simulink model "Model1"  (R2015b)
settings: Solver=ode45  StartTime=0.0  StopTime=4  RelTol=1e-6
undefined symbols (not defined in the file): B_f, B_w, g, J_f, J_w, l_f, l_w, m_f, m_w
settings Model: Creator=USUARIO  LastModifiedBy=USUARIO
settings DataIOCC: LimitDataPoints=off  SaveFormat=Array
settings DebuggingCC: SolverPrmCheckMsg=warning
settings HardwareCC: ProdBitPerPointer=32  ProdLargestAtomicFloat=None  ProdIntDivRoundTo=Undefined  ProdEndianess=Unspecified  ProdWordSize=32  ProdHWDeviceType=32-bit Generic
settings GRTTargetCC: GeneratePreprocessorConditionals=Disable all
settings ConfigComp: CovModelRefEnable=Off  CovSFcnEnable=off

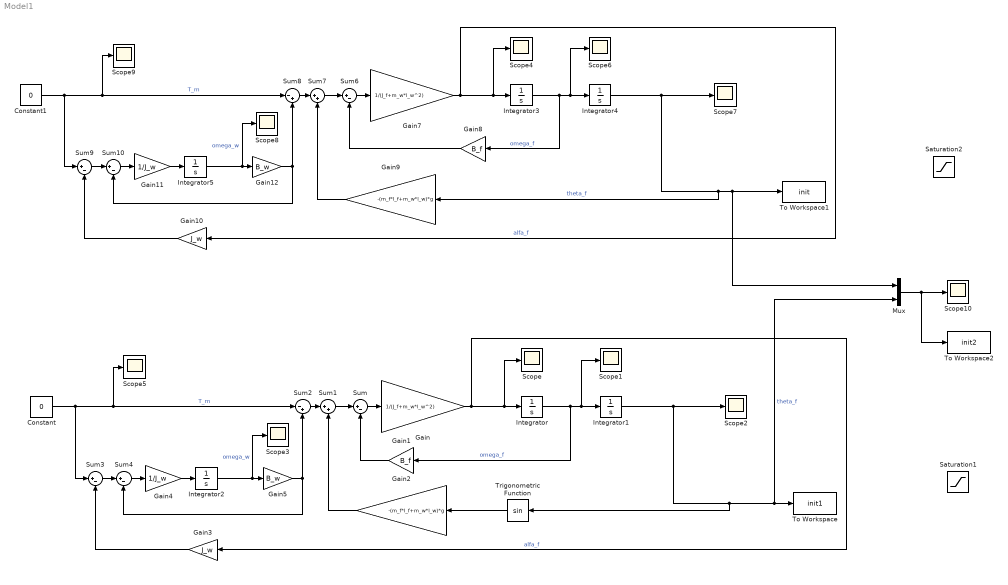
== system Model1 ==
  Constant : Constant  Value=0
  Constant1 : Constant  Value=0
  Gain : Gain  Gain=1/(J_f+m_w*l_w^2)
  Gain1 : Gain  Gain=B_f
  Gain10 : Gain  Gain=J_w
  Gain11 : Gain  Gain=1/J_w
  Gain12 : Gain  Gain=B_w
  Gain2 : Gain  Gain=-(m_f*l_f+m_w*l_w)*g
  Gain3 : Gain  Gain=J_w
  Gain4 : Gain  Gain=1/J_w
  Gain5 : Gain  Gain=B_w
  Gain7 : Gain  Gain=1/(J_f+m_w*l_w^2)
  Gain8 : Gain  Gain=B_f
  Gain9 : Gain  Gain=-(m_f*l_f+m_w*l_w)*g
  Integrator{,2..3,5} (4 alike) : Integrator
  Integrator1 : Integrator  InitialCondition=0.79
  Integrator4 : Integrator  InitialCondition=0.79
  Mux : Mux  Inputs=2
  Saturation1 : Saturate  UpperLimit=6  LowerLimit=-6
  Saturation2 : Saturate  UpperLimit=6  LowerLimit=-6
  Scope{,1..10} (11 alike) : Scope
  Sum{,3..4,6,9..10} (6 alike) : Sum  Inputs=|+-
  Sum1 : Sum  Inputs=|++
  Sum2 : Sum  Inputs=|-+
  Sum7 : Sum  Inputs=|++
  Sum8 : Sum  Inputs=|-+
  To Workspace : ToWorkspace  VariableName=init1  SaveFormat=Timeseries  SampleTime=-1
  To Workspace1 : ToWorkspace  VariableName=init  SaveFormat=Timeseries  SampleTime=-1
  To Workspace2 : ToWorkspace  VariableName=init2  SaveFormat=Timeseries  SampleTime=-1
  Trigonometric Function : Trigonometry
  wires:
  Gain/1 -> Gain3/1, Scope/1, Integrator/1  "alfa_f"
  Integrator/1 -> Gain1/1, Scope1/1, Integrator1/1  "omega_f"
  Sum/1 -> Gain/1
  Sum1/1 -> Sum/1
  Gain1/1 -> Sum/2
  Sum2/1 -> Sum1/1
  Sum4/1 -> Gain4/1
  Gain4/1 -> Integrator2/1
  Gain3/1 -> Sum3/2
  Sum3/1 -> Sum4/1
  Integrator2/1 -> Scope3/1, Gain5/1  "omega_w"
  Gain5/1 -> Sum4/2, Sum2/2
  Constant/1 -> Sum3/1, Scope5/1, Sum2/1  "T_m"
  Integrator1/1 -> Trigonometric Function/1, Mux/2, To Workspace/1, Scope2/1  "theta_f"
  Gain7/1 -> Gain10/1, Scope4/1, Integrator3/1  "alfa_f"
  Integrator3/1 -> Gain8/1, Scope6/1, Integrator4/1  "omega_f"
  Sum6/1 -> Gain7/1
  Sum7/1 -> Sum6/1
  Gain8/1 -> Sum6/2
  Gain9/1 -> Sum7/2
  Sum8/1 -> Sum7/1
  Sum10/1 -> Gain11/1
  Gain11/1 -> Integrator5/1
  Gain10/1 -> Sum9/2
  Sum9/1 -> Sum10/1
  Integrator5/1 -> Scope8/1, Gain12/1  "omega_w"
  Gain12/1 -> Sum10/2, Sum8/2
  Constant1/1 -> Sum9/1, Scope9/1, Sum8/1  "T_m"
  Integrator4/1 -> Gain9/1, Mux/1, To Workspace1/1, Scope7/1  "theta_f"
  Mux/1 -> To Workspace2/1, Scope10/1
  Trigonometric Function/1 -> Gain2/1
  Gain2/1 -> Sum1/2
